simulink model "decentralized_trans"  (R2023b)
settings: Solver=ode45  StartTime=0.0  StopTime=Tf  RelTol=1e-3
undefined symbols (not defined in the file): A_an2, A_an3, Ac_id2, Ac_id3, Ac_mrs2, Ac_mrs3, alpha, b, B_an2, B_an3, Bc_id2, Bc_id3, Bc_mrs2, Bc_mrs3, C2, C3, C_an2, C_an3, C_id2, C_id3, C_opt, Cc_id2, Cc_id3, Cc_mrs2, Cc_mrs3, D_an2, D_an3, Dc_id2, Dc_id3, Dc_mrs2, Dc_mrs3, dx2, dx3, p01, p02, p03, p04, p05, p06, phi02, r_pd1, r_pd2, r_pd3, r_pd4, r_pd5, r_pd6, r_pd_sl1, r_pd_sl2, r_pd_sl3, r_pd_sl4, r_pd_sl5, r_pd_sl6, t1, t2, t3, th, th02, u_max_n1, u_max_n2, u_max_n3 ... (+8)
(part 1 of 2)
settings Model: Creator=lorenzo  LastModifiedBy=lorenzo
settings SolverCC: ZeroCrossControl=DisableAll
settings DebuggingCC: IgnoredZcDiagnostic=none

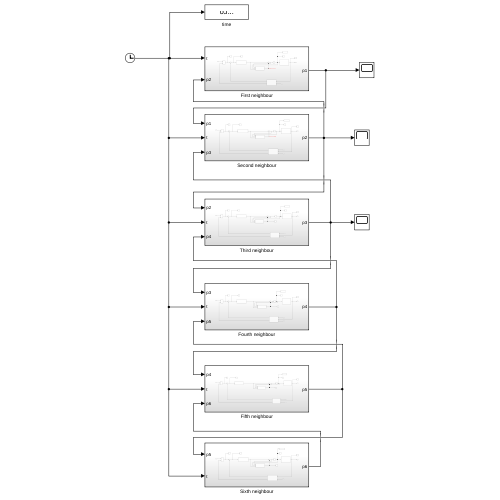
[thumbnail: Simulink's stored preview of the top-level diagram]
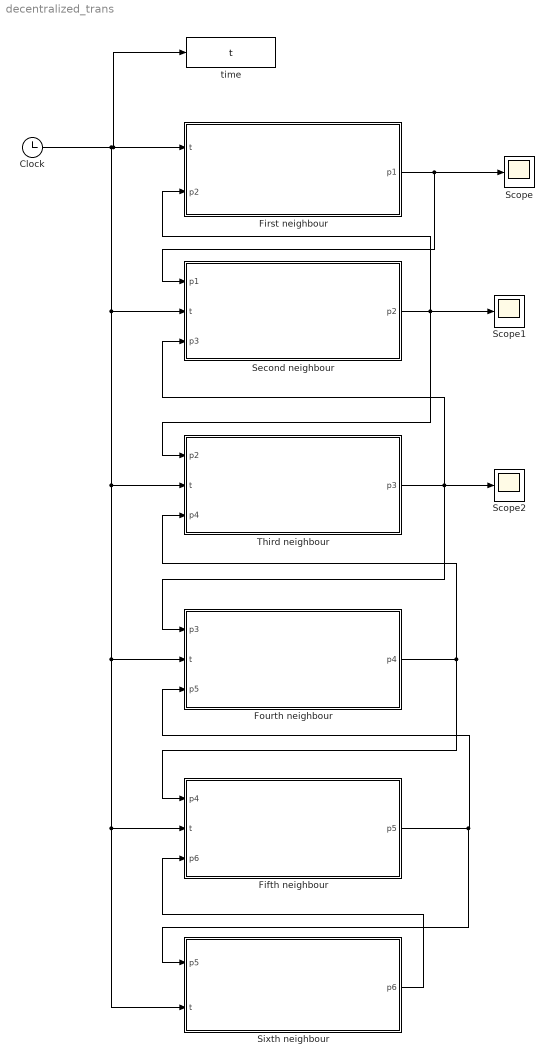
== system decentralized_trans ==
  Clock : Clock
  Fifth neighbour : Subsystem
  First neighbour : Subsystem
  Fourth neighbour : Subsystem
  Scope : Scope
  Scope1 : Scope
  Scope2 : Scope
  Second neighbour : Subsystem
  Sixth neighbour : Subsystem
  Third neighbour : Subsystem
  time : ToWorkspace  VariableName=t  SampleTime=-1
  wires:
  First neighbour/1(p1) -> Second neighbour/1(p1), Scope/1
  Clock/1 -> Sixth neighbour/2(t), Fifth neighbour/2(t), Fourth neighbour/2(t), Third neighbour/2(t), Second neighbour/2(t), First neighbour/1(t), time/1
  Second neighbour/1(p2) -> Scope1/1, First neighbour/2(p2), Third neighbour/1(p2)
  Third neighbour/1(p3) -> Scope2/1, Fourth neighbour/1(p3), Second neighbour/3(p3)
  Fourth neighbour/1(p4) -> Fifth neighbour/1(p4), Third neighbour/3(p4)
  Fifth neighbour/1(p5) -> Sixth neighbour/1(p5), Fourth neighbour/3(p5)
  Sixth neighbour/1(p6) -> Fifth neighbour/3(p6)

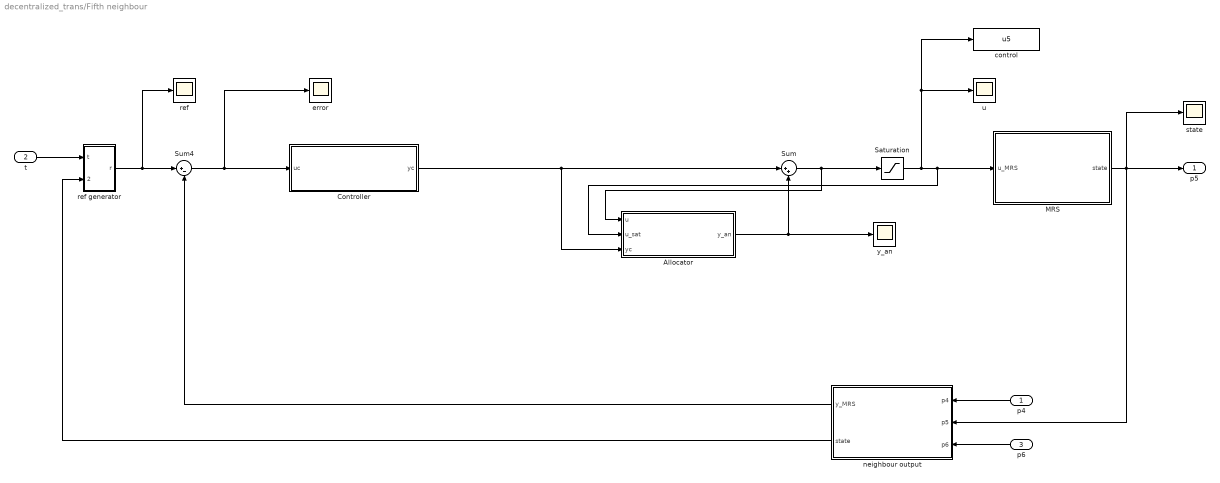
== system decentralized_trans/Fifth neighbour ==
  p4 : Inport
  t : Inport  Port=2
  p6 : Inport  Port=3
  Allocator : Subsystem
  Controller : Subsystem
  MRS : Subsystem
  Saturation : Saturate  UpperLimit=u_max_n5  LowerLimit=-u_max_n5
  Sum : Sum  Inputs=|++
  Sum4 : Sum  Inputs=|+-
  control : ToWorkspace  VariableName=u5  SampleTime=-1
  error : Scope
  neighbour output : Subsystem
  ref : Scope
  ref generator : Subsystem
  state : Scope
  u : Scope
  y_an : Scope
  p5 : Outport
  wires:
  t/1 -> ref generator/1(t)
  Sum4/1 -> error/1, Controller/1(uc)
  MRS/1(state) -> neighbour output/2(p5), state/1, p5/1
  ref generator/1(r) -> ref/1, Sum4/1
  neighbour output/1(y_MRS) -> Sum4/2
  p6/1 -> neighbour output/3(p6)
  neighbour output/2(state) -> ref generator/2(state)
  p4/1 -> neighbour output/1(p4)
  Saturation/1 -> control/1, u/1, Allocator/2(u_sat), MRS/1(u_MRS)
  Sum/1 -> Allocator/1(u), Saturation/1
  Controller/1(yc) -> Allocator/3(yc), Sum/1
  Allocator/1(y_an) -> y_an/1, Sum/2

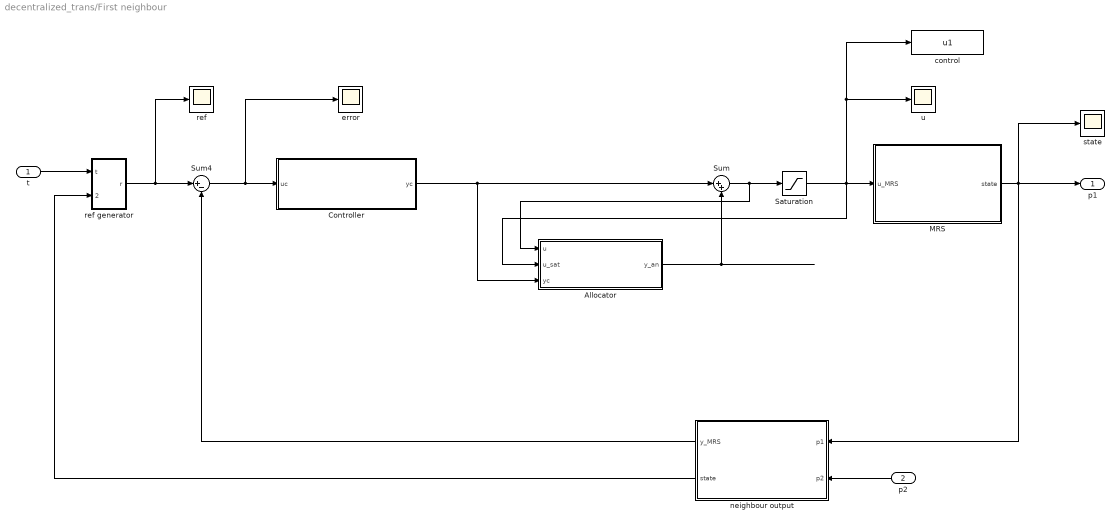
== system decentralized_trans/First neighbour ==
  t : Inport
  p2 : Inport  Port=2
  Allocator : Subsystem
  Controller : Subsystem
  MRS : Subsystem
  Saturation : Saturate  UpperLimit=u_max_n1  LowerLimit=-u_max_n1
  Sum : Sum  Inputs=|++
  Sum4 : Sum  Inputs=|+-
  control : ToWorkspace  VariableName=u1  SampleTime=-1
  error : Scope
  neighbour output : Subsystem
  ref : Scope
  ref generator : Subsystem
  state : Scope
  u : Scope
  p1 : Outport
  wires:
  t/1 -> ref generator/1(t)
  Sum4/1 -> error/1, Controller/1(uc)
  MRS/1(state) -> p1/1, neighbour output/1(p1), state/1
  ref generator/1(r) -> ref/1, Sum4/1
  neighbour output/1(y_MRS) -> Sum4/2
  p2/1 -> neighbour output/2(p2)
  neighbour output/2(state) -> ref generator/2(state)
  Allocator/1(y_an) -> Sum/2
  Sum/1 -> Allocator/1(u), Saturation/1
  Controller/1(yc) -> Allocator/3(yc), Sum/1
  Saturation/1 -> MRS/1(u_MRS), control/1, u/1, Allocator/2(u_sat)

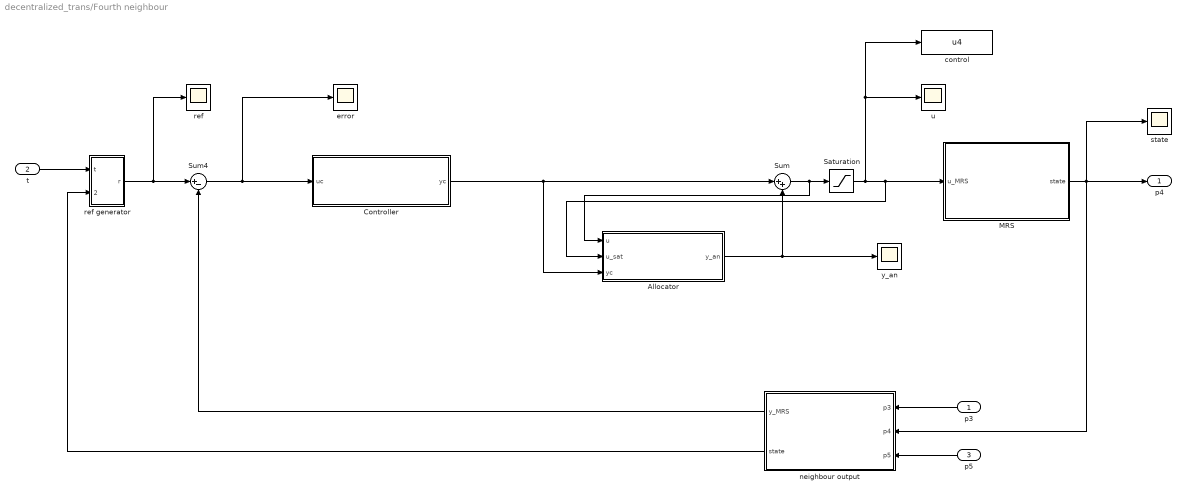
== system decentralized_trans/Fourth neighbour ==
  p3 : Inport
  t : Inport  Port=2
  p5 : Inport  Port=3
  Allocator : Subsystem
  Controller : Subsystem
  MRS : Subsystem
  Saturation : Saturate  UpperLimit=u_max_n4  LowerLimit=-u_max_n4
  Sum : Sum  Inputs=|++
  Sum4 : Sum  Inputs=|+-
  control : ToWorkspace  VariableName=u4  SampleTime=-1
  error : Scope
  neighbour output : Subsystem
  ref : Scope
  ref generator : Subsystem
  state : Scope
  u : Scope
  y_an : Scope
  p4 : Outport
  wires:
  t/1 -> ref generator/1(t)
  Sum4/1 -> error/1, Controller/1(uc)
  MRS/1(state) -> neighbour output/2(p4), state/1, p4/1
  ref generator/1(r) -> ref/1, Sum4/1
  neighbour output/1(y_MRS) -> Sum4/2
  p5/1 -> neighbour output/3(p5)
  neighbour output/2(state) -> ref generator/2(state)
  p3/1 -> neighbour output/1(p3)
  Saturation/1 -> control/1, u/1, Allocator/2(u_sat), MRS/1(u_MRS)
  Sum/1 -> Allocator/1(u), Saturation/1
  Controller/1(yc) -> Allocator/3(yc), Sum/1
  Allocator/1(y_an) -> y_an/1, Sum/2

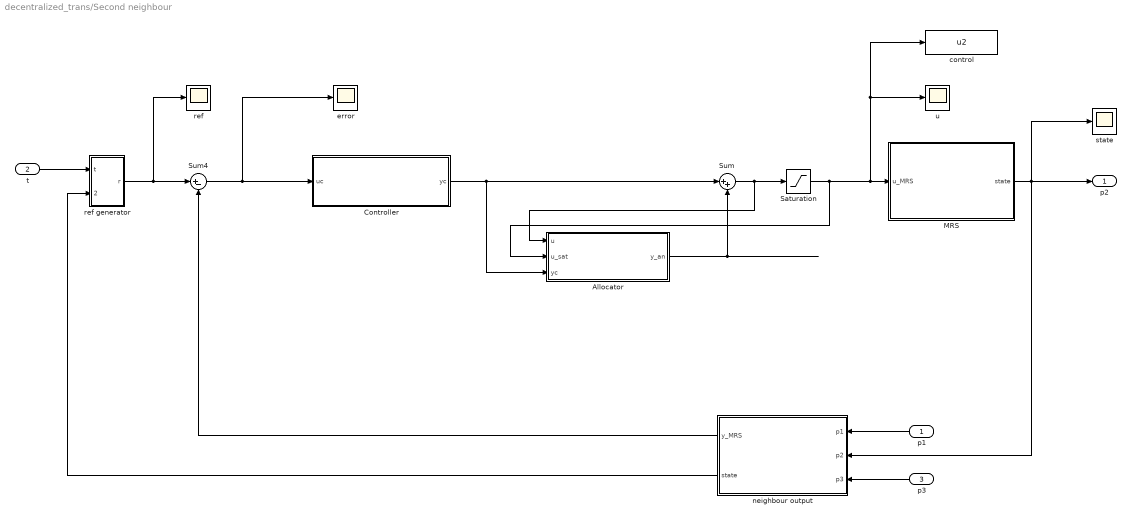
== system decentralized_trans/Second neighbour ==
  p1 : Inport
  t : Inport  Port=2
  p3 : Inport  Port=3
  Allocator : Subsystem
  Controller : Subsystem
  MRS : Subsystem
  Saturation : Saturate  UpperLimit=u_max_n2  LowerLimit=-u_max_n2
  Sum : Sum  Inputs=|++
  Sum4 : Sum  Inputs=|+-
  control : ToWorkspace  VariableName=u2  SampleTime=-1
  error : Scope
  neighbour output : Subsystem
  ref : Scope
  ref generator : Subsystem
  state : Scope
  u : Scope
  p2 : Outport
  wires:
  t/1 -> ref generator/1(t)
  Sum4/1 -> error/1, Controller/1(uc)
  MRS/1(state) -> neighbour output/2(p2), state/1, p2/1
  ref generator/1(r) -> ref/1, Sum4/1
  neighbour output/1(y_MRS) -> Sum4/2
  p3/1 -> neighbour output/3(p3)
  neighbour output/2(state) -> ref generator/2(state)
  p1/1 -> neighbour output/1(p1)
  Allocator/1(y_an) -> Sum/2
  Controller/1(yc) -> Allocator/3(yc), Sum/1
  Sum/1 -> Allocator/1(u), Saturation/1
  Saturation/1 -> MRS/1(u_MRS), control/1, u/1, Allocator/2(u_sat)

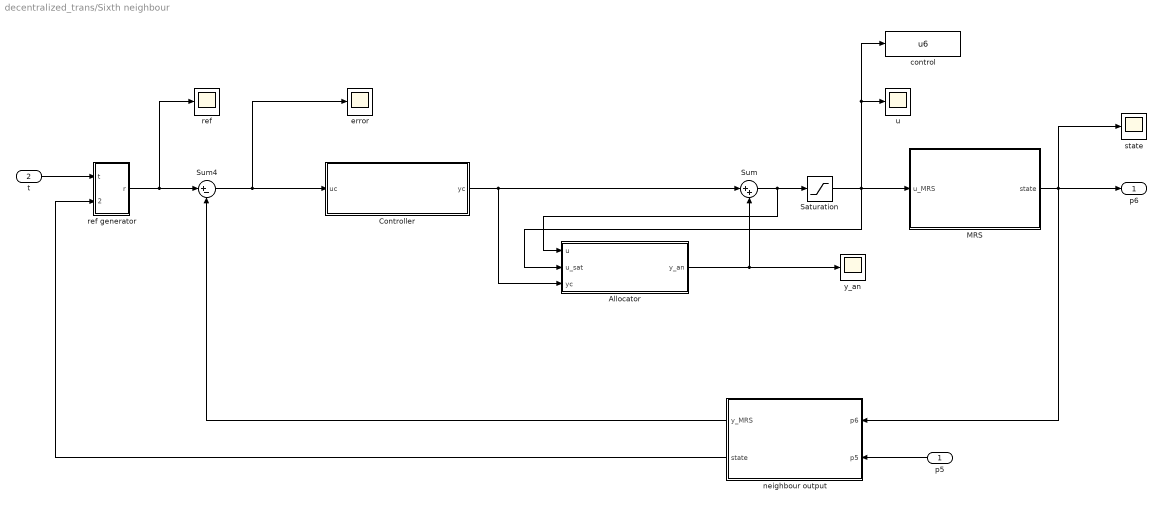
== system decentralized_trans/Sixth neighbour ==
  p5 : Inport
  t : Inport  Port=2
  Allocator : Subsystem
  Controller : Subsystem
  MRS : Subsystem
  Saturation : Saturate  UpperLimit=u_max_n6  LowerLimit=-u_max_n6
  Sum : Sum  Inputs=|++
  Sum4 : Sum  Inputs=|+-
  control : ToWorkspace  VariableName=u6  SampleTime=-1
  error : Scope
  neighbour output : Subsystem
  ref : Scope
  ref generator : Subsystem
  state : Scope
  u : Scope
  y_an : Scope
  p6 : Outport
  wires:
  t/1 -> ref generator/1(t)
  Sum4/1 -> error/1, Controller/1(uc)
  MRS/1(state) -> neighbour output/1(p6), state/1, p6/1
  ref generator/1(r) -> ref/1, Sum4/1
  neighbour output/1(y_MRS) -> Sum4/2
  p5/1 -> neighbour output/2(p5)
  neighbour output/2(state) -> ref generator/2(state)
  Allocator/1(y_an) -> y_an/1, Sum/2
  Controller/1(yc) -> Allocator/3(yc), Sum/1
  Sum/1 -> Allocator/1(u), Saturation/1
  Saturation/1 -> control/1, u/1, Allocator/2(u_sat), MRS/1(u_MRS)

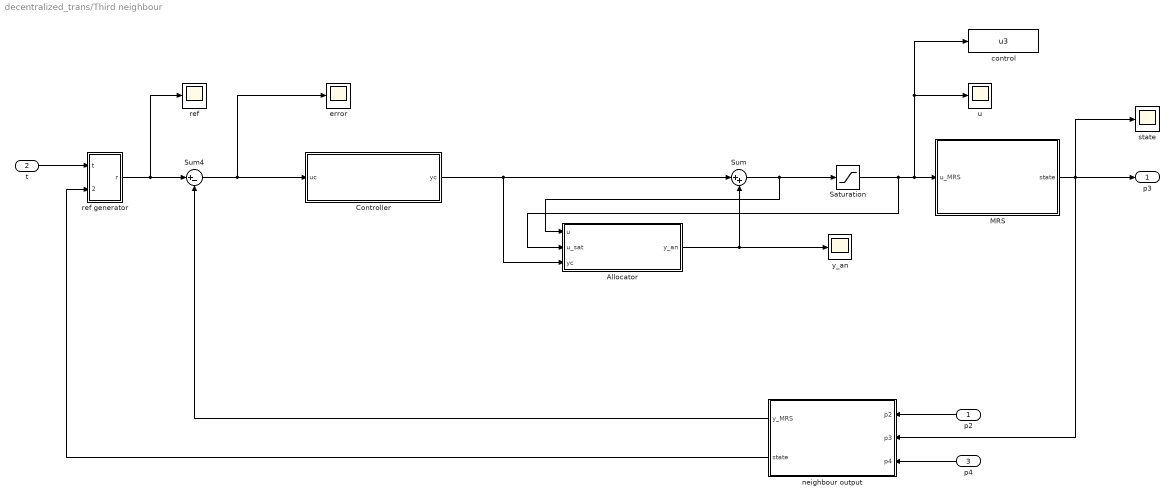
== system decentralized_trans/Third neighbour ==
  p2 : Inport
  t : Inport  Port=2
  p4 : Inport  Port=3
  Allocator : Subsystem
  Controller : Subsystem
  MRS : Subsystem
  Saturation : Saturate  UpperLimit=u_max_n3  LowerLimit=-u_max_n3
  Sum : Sum  Inputs=|++
  Sum4 : Sum  Inputs=|+-
  control : ToWorkspace  VariableName=u3  SampleTime=-1
  error : Scope
  neighbour output : Subsystem
  ref : Scope
  ref generator : Subsystem
  state : Scope
  u : Scope
  y_an : Scope
  p3 : Outport
  wires:
  t/1 -> ref generator/1(t)
  Sum4/1 -> error/1, Controller/1(uc)
  MRS/1(state) -> neighbour output/2(p3), state/1, p3/1
  ref generator/1(r) -> ref/1, Sum4/1
  neighbour output/1(y_MRS) -> Sum4/2
  p4/1 -> neighbour output/3(p4)
  neighbour output/2(state) -> ref generator/2(state)
  p2/1 -> neighbour output/1(p2)
  Saturation/1 -> MRS/1(u_MRS), control/1, u/1, Allocator/2(u_sat)
  Sum/1 -> Allocator/1(u), Saturation/1
  Controller/1(yc) -> Allocator/3(yc), Sum/1
  Allocator/1(y_an) -> y_an/1, Sum/2

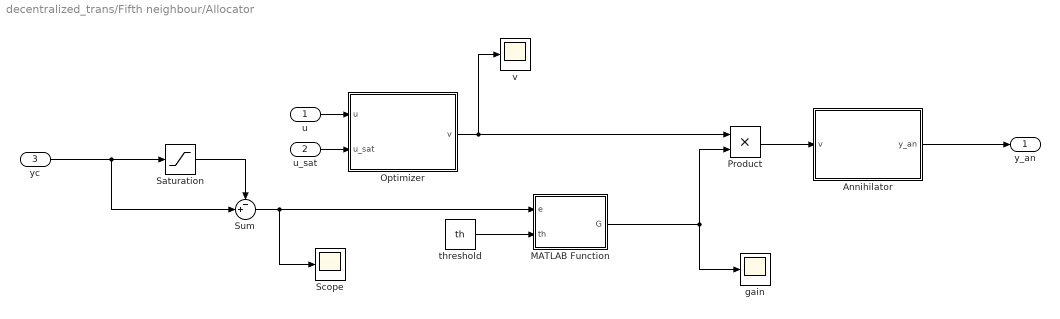
== system decentralized_trans/Fifth neighbour/Allocator ==
  u : Inport
  u_sat : Inport  Port=2
  yc : Inport  Port=3
  Annihilator : Subsystem
  MATLAB Function : MATLAB Function  TreatAsAtomicUnit=on
  Optimizer : Subsystem
  Product : Product
  Saturation : Saturate  UpperLimit=u_max_n5  LowerLimit=-u_max_n5
  Scope : Scope
  Sum : Sum  Inputs=-+|
  gain : Scope
  threshold : Constant  Value=th
  v : Scope
  y_an : Outport
  wires:
  threshold/1 -> MATLAB Function/2(th)
  Optimizer/1(v) -> Product/1, v/1
  u_sat/1 -> Optimizer/2(u_sat)
  MATLAB Function/1(G) -> gain/1, Product/2
  u/1 -> Optimizer/1(u)
  Annihilator/1(y_an) -> y_an/1
  Product/1 -> Annihilator/1(v)
  Saturation/1 -> Sum/1
  Sum/1 -> Scope/1, MATLAB Function/1(e)
  yc/1 -> Sum/2, Saturation/1

== system decentralized_trans/Fifth neighbour/Controller ==
  uc : Inport
  Clock1 : Clock
  Controller formation : Subsystem
  Controller line follow : Subsystem
  MATLAB Function : MATLAB Function  TreatAsAtomicUnit=on
  MATLAB Function1 : MATLAB Function  TreatAsAtomicUnit=on
  Scope : Scope
  t1 : Constant  Value=t1  VectorParams1D=off
  t2 : Constant  Value=t2  VectorParams1D=off
  t3 : Constant  Value=t3  VectorParams1D=off
  yc : Outport
  wires:
  uc/1 -> Controller formation/1(uc), Controller line follow/1(uc)
  Clock1/1 -> MATLAB Function1/1(t), MATLAB Function/2(t)
  Controller line follow/1(u) -> MATLAB Function/1(u_lf)
  Controller formation/1(u) -> MATLAB Function/3(u_f)
  t1/1 -> MATLAB Function1/2(t1), MATLAB Function/4(t1)
  t3/1 -> MATLAB Function1/4(t3), MATLAB Function/6(t3)
  MATLAB Function/1(yc) -> yc/1
  t2/1 -> MATLAB Function1/3(t2), MATLAB Function/5(t2)
  MATLAB Function1/1(y) -> Scope/1, Controller line follow/2(y), Controller formation/2(y)

== system decentralized_trans/Fifth neighbour/MRS ==
  u_MRS : Inport
  Constant : Constant  Value=b
  Integrator : Integrator  InitialCondition=p05
  Integrator1 : Integrator  InitialCondition=th02
  Integrator2 : Integrator  InitialCondition=phi02
  MATLAB Function : MATLAB Function  TreatAsAtomicUnit=on
  Scope : Scope
  Scope1 : Scope
  theta : ToWorkspace  VariableName=theta5  SampleTime=-1
  y : ToWorkspace  VariableName=y5  SampleTime=-1
  state : Outport
  wires:
  u_MRS/1 -> MATLAB Function/1(u)
  Constant/1 -> MATLAB Function/2(b)
  MATLAB Function/2(dth) -> Integrator1/1
  MATLAB Function/1(dp) -> Integrator/1
  Integrator1/1 -> MATLAB Function/3(th), Scope/1, theta/1
  MATLAB Function/3(dphi) -> Integrator2/1
  Integrator2/1 -> Scope1/1, MATLAB Function/4(phi)
  Integrator/1 -> y/1, state/1

== system decentralized_trans/Fifth neighbour/neighbour output ==
  p4 : Inport
  p5 : Inport  Port=2
  p6 : Inport  Port=3
  C : Gain  Gain=C3  Multiplication=Matrix(K*u) (u vector)
  C_id : Gain  Gain=C_id3  Multiplication=Matrix(K*u) (u vector)
  Clock : Clock
  MATLAB Function : MATLAB Function  TreatAsAtomicUnit=on
  MATLAB Function1 : MATLAB Function  TreatAsAtomicUnit=on
  t1 : Constant  Value=t1  VectorParams1D=off
  t2 : Constant  Value=t2  VectorParams1D=off
  t3 : Constant  Value=t3  VectorParams1D=off
  y_MRS : Outport
  state : Outport  Port=2
  wires:
  t2/1 -> MATLAB Function1/5(t2)
  C/1 -> MATLAB Function1/3(y_f)
  Clock/1 -> MATLAB Function1/2(t)
  t3/1 -> MATLAB Function1/6(t3)
  C_id/1 -> MATLAB Function1/1(y_lf)
  MATLAB Function1/1(y_MRS) -> y_MRS/1
  t1/1 -> MATLAB Function1/4(t1)
  MATLAB Function/1(yn) -> state/1, C/1, C_id/1
  p6/1 -> MATLAB Function/3(y3)
  p5/1 -> MATLAB Function/2(y2)
  p4/1 -> MATLAB Function/1(y1)

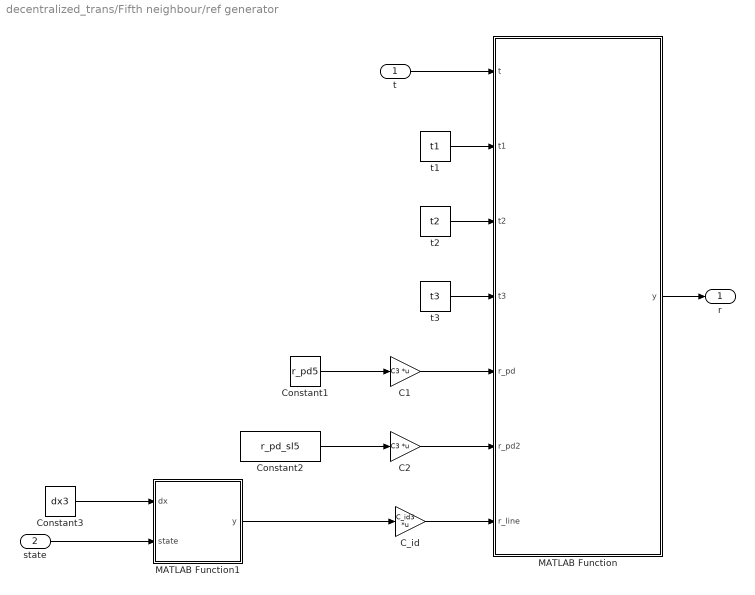
== system decentralized_trans/Fifth neighbour/ref generator ==
  t : Inport
  state : Inport  Port=2
  C1 : Gain  Gain=C3  Multiplication=Matrix(K*u) (u vector)
  C2 : Gain  Gain=C3  Multiplication=Matrix(K*u) (u vector)
  C_id : Gain  Gain=C_id3  Multiplication=Matrix(K*u) (u vector)
  Constant1 : Constant  Value=r_pd5  VectorParams1D=off
  Constant2 : Constant  Value=r_pd_sl5  VectorParams1D=off
  Constant3 : Constant  Value=dx3
  MATLAB Function : MATLAB Function  TreatAsAtomicUnit=on
  MATLAB Function1 : MATLAB Function  TreatAsAtomicUnit=on
  t1 : Constant  Value=t1  VectorParams1D=off
  t2 : Constant  Value=t2  VectorParams1D=off
  t3 : Constant  Value=t3  VectorParams1D=off
  r : Outport
  wires:
  t/1 -> MATLAB Function/1(t)
  t1/1 -> MATLAB Function/2(t1)
  t2/1 -> MATLAB Function/3(t2)
  t3/1 -> MATLAB Function/4(t3)
  Constant2/1 -> C2/1
  C2/1 -> MATLAB Function/6(r_pd2)
  Constant1/1 -> C1/1
  C1/1 -> MATLAB Function/5(r_pd)
  C_id/1 -> MATLAB Function/7(r_line)
  MATLAB Function/1(y) -> r/1
  Constant3/1 -> MATLAB Function1/1(dx)
  state/1 -> MATLAB Function1/2(state)
  MATLAB Function1/1(y) -> C_id/1

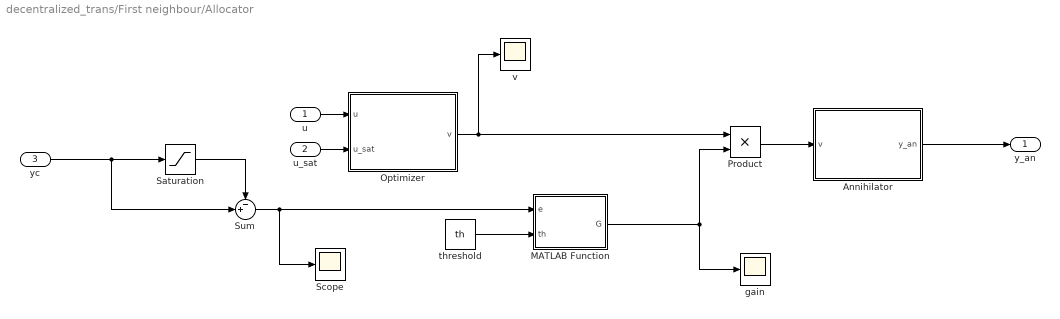
== system decentralized_trans/First neighbour/Allocator ==
  u : Inport
  u_sat : Inport  Port=2
  yc : Inport  Port=3
  Annihilator : Subsystem
  MATLAB Function : MATLAB Function  TreatAsAtomicUnit=on
  Optimizer : Subsystem
  Product : Product
  Saturation : Saturate  UpperLimit=u_max_n1  LowerLimit=-u_max_n1
  Scope : Scope
  Sum : Sum  Inputs=-+|
  gain : Scope
  threshold : Constant  Value=th
  v : Scope
  y_an : Outport
  wires:
  threshold/1 -> MATLAB Function/2(th)
  Optimizer/1(v) -> Product/1, v/1
  u_sat/1 -> Optimizer/2(u_sat)
  MATLAB Function/1(G) -> gain/1, Product/2
  u/1 -> Optimizer/1(u)
  Annihilator/1(y_an) -> y_an/1
  Product/1 -> Annihilator/1(v)
  Saturation/1 -> Sum/1
  Sum/1 -> Scope/1, MATLAB Function/1(e)
  yc/1 -> Sum/2, Saturation/1

== system decentralized_trans/First neighbour/Controller ==
  uc : Inport
  Clock1 : Clock
  Controller formation : Subsystem
  Controller line follow : Subsystem
  MATLAB Function : MATLAB Function  TreatAsAtomicUnit=on
  MATLAB Function1 : MATLAB Function  TreatAsAtomicUnit=on
  Scope : Scope
  t1 : Constant  Value=t1  VectorParams1D=off
  t2 : Constant  Value=t2  VectorParams1D=off
  t3 : Constant  Value=t3  VectorParams1D=off
  yc : Outport
  wires:
  uc/1 -> Controller formation/1(uc), Controller line follow/1(uc)
  Clock1/1 -> MATLAB Function1/1(t), MATLAB Function/2(t)
  Controller line follow/1(u) -> MATLAB Function/1(u_lf)
  Controller formation/1(u) -> MATLAB Function/3(u_f)
  t1/1 -> MATLAB Function1/2(t1), MATLAB Function/4(t1)
  t3/1 -> MATLAB Function1/4(t3), MATLAB Function/6(t3)
  MATLAB Function/1(yc) -> yc/1
  t2/1 -> MATLAB Function1/3(t2), MATLAB Function/5(t2)
  MATLAB Function1/1(y) -> Scope/1, Controller line follow/2(y), Controller formation/2(y)

== system decentralized_trans/First neighbour/MRS ==
  u_MRS : Inport
  Constant : Constant  Value=b
  Integrator : Integrator  InitialCondition=p01
  Integrator1 : Integrator  InitialCondition=th02
  Integrator2 : Integrator  InitialCondition=phi02
  MATLAB Function : MATLAB Function  TreatAsAtomicUnit=on
  Scope : Scope
  Scope1 : Scope
  theta : ToWorkspace  VariableName=theta1  SampleTime=-1
  y : ToWorkspace  VariableName=y1  SampleTime=-1
  state : Outport
  wires:
  u_MRS/1 -> MATLAB Function/1(u)
  Constant/1 -> MATLAB Function/2(b)
  MATLAB Function/2(dth) -> Integrator1/1
  MATLAB Function/1(dp) -> Integrator/1
  Integrator1/1 -> MATLAB Function/3(th), Scope/1, theta/1
  MATLAB Function/3(dphi) -> Integrator2/1
  Integrator2/1 -> Scope1/1, MATLAB Function/4(phi)
  Integrator/1 -> y/1, state/1

== system decentralized_trans/First neighbour/neighbour output ==
  p1 : Inport
  p2 : Inport  Port=2
  C : Gain  Gain=C2  Multiplication=Matrix(K*u) (u vector)
  C_id : Gain  Gain=C_id2  Multiplication=Matrix(K*u) (u vector)
  Clock : Clock
  MATLAB Function : MATLAB Function  TreatAsAtomicUnit=on
  MATLAB Function1 : MATLAB Function  TreatAsAtomicUnit=on
  t1 : Constant  Value=t1  VectorParams1D=off
  t2 : Constant  Value=t2  VectorParams1D=off
  t3 : Constant  Value=t3  VectorParams1D=off
  y_MRS : Outport
  state : Outport  Port=2
  wires:
  t2/1 -> MATLAB Function1/5(t2)
  C/1 -> MATLAB Function1/3(y_f)
  Clock/1 -> MATLAB Function1/2(t)
  t3/1 -> MATLAB Function1/6(t3)
  C_id/1 -> MATLAB Function1/1(y_lf)
  MATLAB Function1/1(y_MRS) -> y_MRS/1
  t1/1 -> MATLAB Function1/4(t1)
  p1/1 -> MATLAB Function/1(y1)
  p2/1 -> MATLAB Function/2(y2)
  MATLAB Function/1(yn) -> state/1, C/1, C_id/1

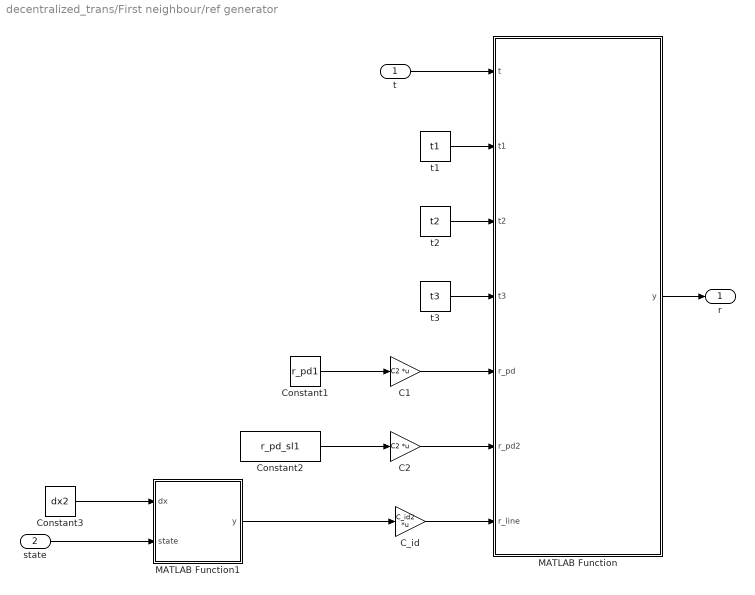
== system decentralized_trans/First neighbour/ref generator ==
  t : Inport
  state : Inport  Port=2
  C1 : Gain  Gain=C2  Multiplication=Matrix(K*u) (u vector)
  C2 : Gain  Gain=C2  Multiplication=Matrix(K*u) (u vector)
  C_id : Gain  Gain=C_id2  Multiplication=Matrix(K*u) (u vector)
  Constant1 : Constant  Value=r_pd1  VectorParams1D=off
  Constant2 : Constant  Value=r_pd_sl1  VectorParams1D=off
  Constant3 : Constant  Value=dx2
  MATLAB Function : MATLAB Function  TreatAsAtomicUnit=on
  MATLAB Function1 : MATLAB Function  TreatAsAtomicUnit=on
  t1 : Constant  Value=t1  VectorParams1D=off
  t2 : Constant  Value=t2  VectorParams1D=off
  t3 : Constant  Value=t3  VectorParams1D=off
  r : Outport
  wires:
  t/1 -> MATLAB Function/1(t)
  t1/1 -> MATLAB Function/2(t1)
  t2/1 -> MATLAB Function/3(t2)
  t3/1 -> MATLAB Function/4(t3)
  Constant2/1 -> C2/1
  C2/1 -> MATLAB Function/6(r_pd2)
  Constant1/1 -> C1/1
  C1/1 -> MATLAB Function/5(r_pd)
  C_id/1 -> MATLAB Function/7(r_line)
  MATLAB Function/1(y) -> r/1
  Constant3/1 -> MATLAB Function1/1(dx)
  state/1 -> MATLAB Function1/2(state)
  MATLAB Function1/1(y) -> C_id/1

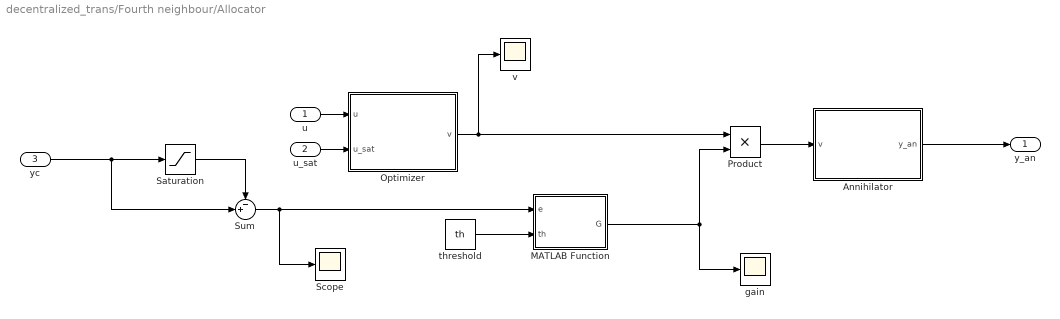
== system decentralized_trans/Fourth neighbour/Allocator ==
  u : Inport
  u_sat : Inport  Port=2
  yc : Inport  Port=3
  Annihilator : Subsystem
  MATLAB Function : MATLAB Function  TreatAsAtomicUnit=on
  Optimizer : Subsystem
  Product : Product
  Saturation : Saturate  UpperLimit=u_max_n4  LowerLimit=-u_max_n4
  Scope : Scope
  Sum : Sum  Inputs=-+|
  gain : Scope
  threshold : Constant  Value=th
  v : Scope
  y_an : Outport
  wires:
  threshold/1 -> MATLAB Function/2(th)
  Optimizer/1(v) -> Product/1, v/1
  u_sat/1 -> Optimizer/2(u_sat)
  MATLAB Function/1(G) -> gain/1, Product/2
  u/1 -> Optimizer/1(u)
  Annihilator/1(y_an) -> y_an/1
  Product/1 -> Annihilator/1(v)
  Saturation/1 -> Sum/1
  Sum/1 -> Scope/1, MATLAB Function/1(e)
  yc/1 -> Sum/2, Saturation/1

== system decentralized_trans/Fourth neighbour/Controller ==
  uc : Inport
  Clock1 : Clock
  Controller formation : Subsystem
  Controller line follow : Subsystem
  MATLAB Function : MATLAB Function  TreatAsAtomicUnit=on
  MATLAB Function1 : MATLAB Function  TreatAsAtomicUnit=on
  Scope : Scope
  t1 : Constant  Value=t1  VectorParams1D=off
  t2 : Constant  Value=t2  VectorParams1D=off
  t3 : Constant  Value=t3  VectorParams1D=off
  yc : Outport
  wires:
  uc/1 -> Controller formation/1(uc), Controller line follow/1(uc)
  Clock1/1 -> MATLAB Function1/1(t), MATLAB Function/2(t)
  Controller line follow/1(u) -> MATLAB Function/1(u_lf)
  Controller formation/1(u) -> MATLAB Function/3(u_f)
  t1/1 -> MATLAB Function1/2(t1), MATLAB Function/4(t1)
  t3/1 -> MATLAB Function1/4(t3), MATLAB Function/6(t3)
  MATLAB Function/1(yc) -> yc/1
  t2/1 -> MATLAB Function1/3(t2), MATLAB Function/5(t2)
  MATLAB Function1/1(y) -> Scope/1, Controller line follow/2(y), Controller formation/2(y)

== system decentralized_trans/Fourth neighbour/MRS ==
  u_MRS : Inport
  Constant : Constant  Value=b
  Integrator : Integrator  InitialCondition=p04
  Integrator1 : Integrator  InitialCondition=th02
  Integrator2 : Integrator  InitialCondition=phi02
  MATLAB Function : MATLAB Function  TreatAsAtomicUnit=on
  Scope : Scope
  Scope1 : Scope
  theta : ToWorkspace  VariableName=theta4  SampleTime=-1
  y : ToWorkspace  VariableName=y4  SampleTime=-1
  state : Outport
  wires:
  u_MRS/1 -> MATLAB Function/1(u)
  Constant/1 -> MATLAB Function/2(b)
  MATLAB Function/2(dth) -> Integrator1/1
  MATLAB Function/1(dp) -> Integrator/1
  Integrator1/1 -> MATLAB Function/3(th), Scope/1, theta/1
  MATLAB Function/3(dphi) -> Integrator2/1
  Integrator2/1 -> Scope1/1, MATLAB Function/4(phi)
  Integrator/1 -> y/1, state/1

== system decentralized_trans/Fourth neighbour/neighbour output ==
  p3 : Inport
  p4 : Inport  Port=2
  p5 : Inport  Port=3
  C : Gain  Gain=C3  Multiplication=Matrix(K*u) (u vector)
  C_id : Gain  Gain=C_id3  Multiplication=Matrix(K*u) (u vector)
  Clock : Clock
  MATLAB Function : MATLAB Function  TreatAsAtomicUnit=on
  MATLAB Function1 : MATLAB Function  TreatAsAtomicUnit=on
  t1 : Constant  Value=t1  VectorParams1D=off
  t2 : Constant  Value=t2  VectorParams1D=off
  t3 : Constant  Value=t3  VectorParams1D=off
  y_MRS : Outport
  state : Outport  Port=2
  wires:
  t2/1 -> MATLAB Function1/5(t2)
  C/1 -> MATLAB Function1/3(y_f)
  Clock/1 -> MATLAB Function1/2(t)
  t3/1 -> MATLAB Function1/6(t3)
  C_id/1 -> MATLAB Function1/1(y_lf)
  MATLAB Function1/1(y_MRS) -> y_MRS/1
  t1/1 -> MATLAB Function1/4(t1)
  MATLAB Function/1(yn) -> state/1, C/1, C_id/1
  p5/1 -> MATLAB Function/3(y3)
  p4/1 -> MATLAB Function/2(y2)
  p3/1 -> MATLAB Function/1(y1)

== system decentralized_trans/Fourth neighbour/ref generator ==
  t : Inport
  state : Inport  Port=2
  C1 : Gain  Gain=C3  Multiplication=Matrix(K*u) (u vector)
  C2 : Gain  Gain=C3  Multiplication=Matrix(K*u) (u vector)
  C_id : Gain  Gain=C_id3  Multiplication=Matrix(K*u) (u vector)
  Constant1 : Constant  Value=r_pd4  VectorParams1D=off
  Constant2 : Constant  Value=r_pd_sl4  VectorParams1D=off
  Constant3 : Constant  Value=dx3
  MATLAB Function : MATLAB Function  TreatAsAtomicUnit=on
  MATLAB Function1 : MATLAB Function  TreatAsAtomicUnit=on
  t1 : Constant  Value=t1  VectorParams1D=off
  t2 : Constant  Value=t2  VectorParams1D=off
  t3 : Constant  Value=t3  VectorParams1D=off
  r : Outport
  wires:
  t/1 -> MATLAB Function/1(t)
  t1/1 -> MATLAB Function/2(t1)
  t2/1 -> MATLAB Function/3(t2)
  t3/1 -> MATLAB Function/4(t3)
  Constant2/1 -> C2/1
  C2/1 -> MATLAB Function/6(r_pd2)
  Constant1/1 -> C1/1
  C1/1 -> MATLAB Function/5(r_pd)
  C_id/1 -> MATLAB Function/7(r_line)
  MATLAB Function/1(y) -> r/1
  Constant3/1 -> MATLAB Function1/1(dx)
  state/1 -> MATLAB Function1/2(state)
  MATLAB Function1/1(y) -> C_id/1

== system decentralized_trans/Second neighbour/Allocator ==
  u : Inport
  u_sat : Inport  Port=2
  yc : Inport  Port=3
  Annihilator : Subsystem
  MATLAB Function : MATLAB Function  TreatAsAtomicUnit=on
  Optimizer : Subsystem
  Product : Product
  Saturation : Saturate  UpperLimit=u_max_n2  LowerLimit=-u_max_n2
  Scope : Scope
  Sum : Sum  Inputs=-+|
  gain : Scope
  threshold : Constant  Value=th
  v : Scope
  y_an : Outport
  wires:
  threshold/1 -> MATLAB Function/2(th)
  Optimizer/1(v) -> Product/1, v/1
  u_sat/1 -> Optimizer/2(u_sat)
  MATLAB Function/1(G) -> gain/1, Product/2
  u/1 -> Optimizer/1(u)
  Annihilator/1(y_an) -> y_an/1
  Product/1 -> Annihilator/1(v)
  Saturation/1 -> Sum/1
  Sum/1 -> Scope/1, MATLAB Function/1(e)
  yc/1 -> Sum/2, Saturation/1

== system decentralized_trans/Second neighbour/Controller ==
  uc : Inport
  Clock1 : Clock
  Controller formation : Subsystem
  Controller line follow : Subsystem
  MATLAB Function : MATLAB Function  TreatAsAtomicUnit=on
  MATLAB Function1 : MATLAB Function  TreatAsAtomicUnit=on
  Scope : Scope
  t1 : Constant  Value=t1  VectorParams1D=off
  t2 : Constant  Value=t2  VectorParams1D=off
  t3 : Constant  Value=t3  VectorParams1D=off
  yc : Outport
  wires:
  uc/1 -> Controller formation/1(uc), Controller line follow/1(uc)
  Clock1/1 -> MATLAB Function1/1(t), MATLAB Function/2(t)
  Controller line follow/1(u) -> MATLAB Function/1(u_lf)
  Controller formation/1(u) -> MATLAB Function/3(u_f)
  t1/1 -> MATLAB Function1/2(t1), MATLAB Function/4(t1)
  t3/1 -> MATLAB Function1/4(t3), MATLAB Function/6(t3)
  MATLAB Function/1(yc) -> yc/1
  t2/1 -> MATLAB Function1/3(t2), MATLAB Function/5(t2)
  MATLAB Function1/1(y) -> Scope/1, Controller line follow/2(y), Controller formation/2(y)

== system decentralized_trans/Second neighbour/MRS ==
  u_MRS : Inport
  Constant : Constant  Value=b
  Integrator : Integrator  InitialCondition=p02
  Integrator1 : Integrator  InitialCondition=th02
  Integrator2 : Integrator  InitialCondition=phi02
  MATLAB Function : MATLAB Function  TreatAsAtomicUnit=on
  Scope : Scope
  Scope1 : Scope
  theta : ToWorkspace  VariableName=theta2  SampleTime=-1
  y : ToWorkspace  VariableName=y2  SampleTime=-1
  state : Outport
  wires:
  u_MRS/1 -> MATLAB Function/1(u)
  Constant/1 -> MATLAB Function/2(b)
  MATLAB Function/2(dth) -> Integrator1/1
  MATLAB Function/1(dp) -> Integrator/1
  Integrator1/1 -> MATLAB Function/3(th), Scope/1, theta/1
  MATLAB Function/3(dphi) -> Integrator2/1
  Integrator2/1 -> Scope1/1, MATLAB Function/4(phi)
  Integrator/1 -> y/1, state/1

== system decentralized_trans/Second neighbour/neighbour output ==
  p1 : Inport
  p2 : Inport  Port=2
  p3 : Inport  Port=3
  C : Gain  Gain=C3  Multiplication=Matrix(K*u) (u vector)
  C_id : Gain  Gain=C_id3  Multiplication=Matrix(K*u) (u vector)
  Clock : Clock
  MATLAB Function : MATLAB Function  TreatAsAtomicUnit=on
  MATLAB Function1 : MATLAB Function  TreatAsAtomicUnit=on
  t1 : Constant  Value=t1  VectorParams1D=off
  t2 : Constant  Value=t2  VectorParams1D=off
  t3 : Constant  Value=t3  VectorParams1D=off
  y_MRS : Outport
  state : Outport  Port=2
  wires:
  t2/1 -> MATLAB Function1/5(t2)
  C/1 -> MATLAB Function1/3(y_f)
  Clock/1 -> MATLAB Function1/2(t)
  t3/1 -> MATLAB Function1/6(t3)
  C_id/1 -> MATLAB Function1/1(y_lf)
  MATLAB Function1/1(y_MRS) -> y_MRS/1
  t1/1 -> MATLAB Function1/4(t1)
  MATLAB Function/1(yn) -> state/1, C/1, C_id/1
  p3/1 -> MATLAB Function/3(y3)
  p2/1 -> MATLAB Function/2(y2)
  p1/1 -> MATLAB Function/1(y1)

== system decentralized_trans/Second neighbour/ref generator ==
  t : Inport
  state : Inport  Port=2
  C1 : Gain  Gain=C3  Multiplication=Matrix(K*u) (u vector)
  C2 : Gain  Gain=C3  Multiplication=Matrix(K*u) (u vector)
  C_id : Gain  Gain=C_id3  Multiplication=Matrix(K*u) (u vector)
  Constant1 : Constant  Value=r_pd2  VectorParams1D=off
  Constant2 : Constant  Value=r_pd_sl2  VectorParams1D=off
  Constant3 : Constant  Value=dx3
  MATLAB Function : MATLAB Function  TreatAsAtomicUnit=on
  MATLAB Function1 : MATLAB Function  TreatAsAtomicUnit=on
  t1 : Constant  Value=t1  VectorParams1D=off
  t2 : Constant  Value=t2  VectorParams1D=off
  t3 : Constant  Value=t3  VectorParams1D=off
  r : Outport
  wires:
  t/1 -> MATLAB Function/1(t)
  t1/1 -> MATLAB Function/2(t1)
  t2/1 -> MATLAB Function/3(t2)
  t3/1 -> MATLAB Function/4(t3)
  Constant2/1 -> C2/1
  C2/1 -> MATLAB Function/6(r_pd2)
  Constant1/1 -> C1/1
  C1/1 -> MATLAB Function/5(r_pd)
  C_id/1 -> MATLAB Function/7(r_line)
  MATLAB Function/1(y) -> r/1
  Constant3/1 -> MATLAB Function1/1(dx)
  state/1 -> MATLAB Function1/2(state)
  MATLAB Function1/1(y) -> C_id/1

== system decentralized_trans/Sixth neighbour/Allocator ==
  u : Inport
  u_sat : Inport  Port=2
  yc : Inport  Port=3
  Annihilator : Subsystem
  MATLAB Function : MATLAB Function  TreatAsAtomicUnit=on
  Optimizer : Subsystem
  Product : Product
  Saturation : Saturate  UpperLimit=u_max_n6  LowerLimit=-u_max_n6
  Scope : Scope
  Sum : Sum  Inputs=-+|
  gain : Scope
  threshold : Constant  Value=th
  v : Scope
  y_an : Outport
  wires:
  threshold/1 -> MATLAB Function/2(th)
  Optimizer/1(v) -> Product/1, v/1
  u_sat/1 -> Optimizer/2(u_sat)
  MATLAB Function/1(G) -> gain/1, Product/2
  u/1 -> Optimizer/1(u)
  Annihilator/1(y_an) -> y_an/1
  Product/1 -> Annihilator/1(v)
  Saturation/1 -> Sum/1
  Sum/1 -> Scope/1, MATLAB Function/1(e)
  yc/1 -> Sum/2, Saturation/1

== system decentralized_trans/Sixth neighbour/Controller ==
  uc : Inport
  Clock1 : Clock
  Controller formation : Subsystem
  Controller line follow : Subsystem
  MATLAB Function : MATLAB Function  TreatAsAtomicUnit=on
  MATLAB Function1 : MATLAB Function  TreatAsAtomicUnit=on
  Scope : Scope
  t1 : Constant  Value=t1  VectorParams1D=off
  t2 : Constant  Value=t2  VectorParams1D=off
  t3 : Constant  Value=t3  VectorParams1D=off
  yc : Outport
  wires:
  uc/1 -> Controller formation/1(uc), Controller line follow/1(uc)
  Clock1/1 -> MATLAB Function1/1(t), MATLAB Function/2(t)
  Controller line follow/1(u) -> MATLAB Function/1(u_lf)
  Controller formation/1(u) -> MATLAB Function/3(u_f)
  t1/1 -> MATLAB Function1/2(t1), MATLAB Function/4(t1)
  t3/1 -> MATLAB Function1/4(t3), MATLAB Function/6(t3)
  MATLAB Function/1(yc) -> yc/1
  t2/1 -> MATLAB Function1/3(t2), MATLAB Function/5(t2)
  MATLAB Function1/1(y) -> Scope/1, Controller line follow/2(y), Controller formation/2(y)

== system decentralized_trans/Sixth neighbour/MRS ==
  u_MRS : Inport
  Constant : Constant  Value=b
  Integrator : Integrator  InitialCondition=p06
  Integrator1 : Integrator  InitialCondition=th02
  Integrator2 : Integrator  InitialCondition=phi02
  MATLAB Function : MATLAB Function  TreatAsAtomicUnit=on
  Scope : Scope
  Scope1 : Scope
  theta : ToWorkspace  VariableName=theta6  SampleTime=-1
  y : ToWorkspace  VariableName=y6  SampleTime=-1
  state : Outport
  wires:
  u_MRS/1 -> MATLAB Function/1(u)
  Constant/1 -> MATLAB Function/2(b)
  MATLAB Function/2(dth) -> Integrator1/1
  MATLAB Function/1(dp) -> Integrator/1
  Integrator1/1 -> MATLAB Function/3(th), Scope/1, theta/1
  MATLAB Function/3(dphi) -> Integrator2/1
  Integrator2/1 -> Scope1/1, MATLAB Function/4(phi)
  Integrator/1 -> y/1, state/1

== system decentralized_trans/Sixth neighbour/neighbour output ==
  p6 : Inport
  p5 : Inport  Port=2
  C : Gain  Gain=C2  Multiplication=Matrix(K*u) (u vector)
  C_id : Gain  Gain=C_id2  Multiplication=Matrix(K*u) (u vector)
  Clock : Clock
  MATLAB Function : MATLAB Function  TreatAsAtomicUnit=on
  MATLAB Function1 : MATLAB Function  TreatAsAtomicUnit=on
  t1 : Constant  Value=t1  VectorParams1D=off
  t2 : Constant  Value=t2  VectorParams1D=off
  t3 : Constant  Value=t3  VectorParams1D=off
  y_MRS : Outport
  state : Outport  Port=2
  wires:
  t2/1 -> MATLAB Function1/5(t2)
  C/1 -> MATLAB Function1/3(y_f)
  Clock/1 -> MATLAB Function1/2(t)
  t3/1 -> MATLAB Function1/6(t3)
  C_id/1 -> MATLAB Function1/1(y_lf)
  MATLAB Function1/1(y_MRS) -> y_MRS/1
  t1/1 -> MATLAB Function1/4(t1)
  MATLAB Function/1(yn) -> state/1, C/1, C_id/1
  p5/1 -> MATLAB Function/1(y1)
  p6/1 -> MATLAB Function/2(y2)

== system decentralized_trans/Sixth neighbour/ref generator ==
  t : Inport
  state : Inport  Port=2
  C1 : Gain  Gain=C2  Multiplication=Matrix(K*u) (u vector)
  C2 : Gain  Gain=C2  Multiplication=Matrix(K*u) (u vector)
  C_id : Gain  Gain=C_id2  Multiplication=Matrix(K*u) (u vector)
  Constant1 : Constant  Value=r_pd6  VectorParams1D=off
  Constant2 : Constant  Value=r_pd_sl6  VectorParams1D=off
  Constant3 : Constant  Value=dx2
  MATLAB Function : MATLAB Function  TreatAsAtomicUnit=on
  MATLAB Function1 : MATLAB Function  TreatAsAtomicUnit=on
  t1 : Constant  Value=t1  VectorParams1D=off
  t2 : Constant  Value=t2  VectorParams1D=off
  t3 : Constant  Value=t3  VectorParams1D=off
  r : Outport
  wires:
  t/1 -> MATLAB Function/1(t)
  t1/1 -> MATLAB Function/2(t1)
  t2/1 -> MATLAB Function/3(t2)
  t3/1 -> MATLAB Function/4(t3)
  Constant2/1 -> C2/1
  C2/1 -> MATLAB Function/6(r_pd2)
  Constant1/1 -> C1/1
  C1/1 -> MATLAB Function/5(r_pd)
  C_id/1 -> MATLAB Function/7(r_line)
  MATLAB Function/1(y) -> r/1
  Constant3/1 -> MATLAB Function1/1(dx)
  state/1 -> MATLAB Function1/2(state)
  MATLAB Function1/1(y) -> C_id/1

== system decentralized_trans/Third neighbour/Allocator ==
  u : Inport
  u_sat : Inport  Port=2
  yc : Inport  Port=3
  Annihilator : Subsystem
  MATLAB Function : MATLAB Function  TreatAsAtomicUnit=on
  Optimizer : Subsystem
  Product : Product
  Saturation : Saturate  UpperLimit=u_max_n3  LowerLimit=-u_max_n3
  Scope : Scope
  Sum : Sum  Inputs=-+|
  gain : Scope
  threshold : Constant  Value=th
  v : Scope
  y_an : Outport
  wires:
  threshold/1 -> MATLAB Function/2(th)
  Optimizer/1(v) -> Product/1, v/1
  u_sat/1 -> Optimizer/2(u_sat)
  MATLAB Function/1(G) -> gain/1, Product/2
  u/1 -> Optimizer/1(u)
  Annihilator/1(y_an) -> y_an/1
  Product/1 -> Annihilator/1(v)
  Saturation/1 -> Sum/1
  Sum/1 -> Scope/1, MATLAB Function/1(e)
  yc/1 -> Sum/2, Saturation/1

== system decentralized_trans/Third neighbour/Controller ==
  uc : Inport
  Clock1 : Clock
  Controller formation : Subsystem
  Controller line follow : Subsystem
  MATLAB Function : MATLAB Function  TreatAsAtomicUnit=on
  MATLAB Function1 : MATLAB Function  TreatAsAtomicUnit=on
  Scope : Scope
  t1 : Constant  Value=t1  VectorParams1D=off
  t2 : Constant  Value=t2  VectorParams1D=off
  t3 : Constant  Value=t3  VectorParams1D=off
  yc : Outport
  wires:
  uc/1 -> Controller formation/1(uc), Controller line follow/1(uc)
  Clock1/1 -> MATLAB Function1/1(t), MATLAB Function/2(t)
  Controller line follow/1(u) -> MATLAB Function/1(u_lf)
  Controller formation/1(u) -> MATLAB Function/3(u_f)
  t1/1 -> MATLAB Function1/2(t1), MATLAB Function/4(t1)
  t3/1 -> MATLAB Function1/4(t3), MATLAB Function/6(t3)
  MATLAB Function/1(yc) -> yc/1
  t2/1 -> MATLAB Function1/3(t2), MATLAB Function/5(t2)
  MATLAB Function1/1(y) -> Scope/1, Controller line follow/2(y), Controller formation/2(y)

== system decentralized_trans/Third neighbour/MRS ==
  u_MRS : Inport
  Constant : Constant  Value=b
  Integrator : Integrator  InitialCondition=p03
  Integrator1 : Integrator  InitialCondition=th02
  Integrator2 : Integrator  InitialCondition=phi02
  MATLAB Function : MATLAB Function  TreatAsAtomicUnit=on
  Scope : Scope
  Scope1 : Scope
  theta : ToWorkspace  VariableName=theta3  SampleTime=-1
  y : ToWorkspace  VariableName=y3  SampleTime=-1
  state : Outport
  wires:
  u_MRS/1 -> MATLAB Function/1(u)
  Constant/1 -> MATLAB Function/2(b)
  MATLAB Function/2(dth) -> Integrator1/1
  MATLAB Function/1(dp) -> Integrator/1
  Integrator1/1 -> MATLAB Function/3(th), Scope/1, theta/1
  MATLAB Function/3(dphi) -> Integrator2/1
  Integrator2/1 -> Scope1/1, MATLAB Function/4(phi)
  Integrator/1 -> y/1, state/1

== system decentralized_trans/Third neighbour/neighbour output ==
  p2 : Inport
  p3 : Inport  Port=2
  p4 : Inport  Port=3
  C : Gain  Gain=C3  Multiplication=Matrix(K*u) (u vector)
  C_id : Gain  Gain=C_id3  Multiplication=Matrix(K*u) (u vector)
  Clock : Clock
  MATLAB Function : MATLAB Function  TreatAsAtomicUnit=on
  MATLAB Function1 : MATLAB Function  TreatAsAtomicUnit=on
  t1 : Constant  Value=t1  VectorParams1D=off
  t2 : Constant  Value=t2  VectorParams1D=off
  t3 : Constant  Value=t3  VectorParams1D=off
  y_MRS : Outport
  state : Outport  Port=2
  wires:
  t2/1 -> MATLAB Function1/5(t2)
  C/1 -> MATLAB Function1/3(y_f)
  Clock/1 -> MATLAB Function1/2(t)
  t3/1 -> MATLAB Function1/6(t3)
  C_id/1 -> MATLAB Function1/1(y_lf)
  MATLAB Function1/1(y_MRS) -> y_MRS/1
  t1/1 -> MATLAB Function1/4(t1)
  MATLAB Function/1(yn) -> state/1, C/1, C_id/1
  p4/1 -> MATLAB Function/3(y3)
  p3/1 -> MATLAB Function/2(y2)
  p2/1 -> MATLAB Function/1(y1)

== system decentralized_trans/Third neighbour/ref generator ==
  t : Inport
  state : Inport  Port=2
  C1 : Gain  Gain=C3  Multiplication=Matrix(K*u) (u vector)
  C2 : Gain  Gain=C3  Multiplication=Matrix(K*u) (u vector)
  C_id : Gain  Gain=C_id3  Multiplication=Matrix(K*u) (u vector)
  Constant1 : Constant  Value=r_pd3  VectorParams1D=off
  Constant2 : Constant  Value=r_pd_sl3  VectorParams1D=off
  Constant3 : Constant  Value=dx3
  MATLAB Function : MATLAB Function  TreatAsAtomicUnit=on
  MATLAB Function1 : MATLAB Function  TreatAsAtomicUnit=on
  t1 : Constant  Value=t1  VectorParams1D=off
  t2 : Constant  Value=t2  VectorParams1D=off
  t3 : Constant  Value=t3  VectorParams1D=off
  r : Outport
  wires:
  t/1 -> MATLAB Function/1(t)
  t1/1 -> MATLAB Function/2(t1)
  t2/1 -> MATLAB Function/3(t2)
  t3/1 -> MATLAB Function/4(t3)
  Constant2/1 -> C2/1
  C2/1 -> MATLAB Function/6(r_pd2)
  Constant1/1 -> C1/1
  C1/1 -> MATLAB Function/5(r_pd)
  C_id/1 -> MATLAB Function/7(r_line)
  MATLAB Function/1(y) -> r/1
  Constant3/1 -> MATLAB Function1/1(dx)
  state/1 -> MATLAB Function1/2(state)
  MATLAB Function1/1(y) -> C_id/1

== system decentralized_trans/Fifth neighbour/Allocator/Annihilator ==
  v : Inport
  A_an : Gain  Gain=A_an3  Multiplication=Matrix(K*u) (u vector)
  B_an : Gain  Gain=B_an3  Multiplication=Matrix(K*u) (u vector)
  C_an : Gain  Gain=C_an3  Multiplication=Matrix(K*u) (u vector)
  D_an : Gain  Gain=D_an3  Multiplication=Matrix(K*u) (u vector)
  Integrator : Integrator  InitialCondition=xan03
  Sum : Sum  Inputs=|++
  Sum1 : Sum  Inputs=++|
  y_an1 : ToWorkspace  VariableName=yan5  SampleTime=-1
  y_an : Outport
  wires:
  Integrator/1 -> C_an/1, A_an/1
  B_an/1 -> Sum/2
  A_an/1 -> Sum/1
  v/1 -> D_an/1, B_an/1
  Sum/1 -> Integrator/1
  C_an/1 -> Sum1/2
  D_an/1 -> Sum1/1
  Sum1/1 -> y_an1/1, y_an/1

== system decentralized_trans/Fifth neighbour/Allocator/Optimizer ==
  u : Inport
  u_sat : Inport  Port=2
  C_opt : Gain  Gain=C_opt  Multiplication=Matrix(K*u) (u vector)
  Constant : Constant  Value=alpha
  Dan : Constant  Value=D_an3  VectorParams1D=off
  Integrator : Integrator  InitialCondition=xopt0
  Scope : Scope
  dx_opt : MATLAB Function  TreatAsAtomicUnit=on
  u_max : Constant  Value=u_max_n5
  v : Outport
  wires:
  dx_opt/1(dx_opt) -> Scope/1, Integrator/1
  C_opt/1 -> v/1
  Constant/1 -> dx_opt/1(alpha)
  Dan/1 -> dx_opt/2(D_an)
  u_max/1 -> dx_opt/3(u_max)
  u/1 -> dx_opt/4(u)
  u_sat/1 -> dx_opt/5(u_sat)
  Integrator/1 -> C_opt/1

== system decentralized_trans/Fifth neighbour/Controller/Controller formation ==
  uc : Inport
  y : Inport  Port=2
  Ac_mrs : Gain  Gain=Ac_mrs3  Multiplication=Matrix(K*u) (u vector)
  Bc_mrs : Gain  Gain=Bc_mrs3  Multiplication=Matrix(K*u) (u vector)
  Cc_mrs : Gain  Gain=Cc_mrs3  Multiplication=Matrix(K*u) (u vector)
  Dc_mrs : Gain  Gain=Dc_mrs3  Multiplication=Matrix(K*u) (u vector)
  Integrator : Integrator  ExternalReset=either  InitialCondition=xc03
  Sum : Sum  Inputs=|++
  Sum1 : Sum  Inputs=++|
  u : Outport
  wires:
  Bc_mrs/1 -> Sum1/1
  Cc_mrs/1 -> Sum/1
  uc/1 -> Bc_mrs/1, Dc_mrs/1
  Integrator/1 -> Ac_mrs/1, Cc_mrs/1
  Dc_mrs/1 -> Sum/2
  Sum/1 -> u/1
  Ac_mrs/1 -> Sum1/2
  Sum1/1 -> Integrator/1
  y/1 -> Integrator/2

== system decentralized_trans/Fifth neighbour/Controller/Controller line follow ==
  uc : Inport
  y : Inport  Port=2
  Ac_id : Gain  Gain=Ac_id3  Multiplication=Matrix(K*u) (u vector)
  Bc_id : Gain  Gain=Bc_id3  Multiplication=Matrix(K*u) (u vector)
  Cc_id : Gain  Gain=Cc_id3  Multiplication=Matrix(K*u) (u vector)
  Dc_id : Gain  Gain=Dc_id3  Multiplication=Matrix(K*u) (u vector)
  Integrator : Integrator  ExternalReset=either  InitialCondition=xc03
  Sum : Sum  Inputs=|++
  Sum1 : Sum  Inputs=++|
  u : Outport
  wires:
  Bc_id/1 -> Sum1/1
  Cc_id/1 -> Sum/1
  uc/1 -> Bc_id/1, Dc_id/1
  Integrator/1 -> Ac_id/1, Cc_id/1
  Dc_id/1 -> Sum/2
  Sum/1 -> u/1
  Ac_id/1 -> Sum1/2
  Sum1/1 -> Integrator/1
  y/1 -> Integrator/2

== system decentralized_trans/First neighbour/Allocator/Annihilator ==
  v : Inport
  A_an : Gain  Gain=A_an2  Multiplication=Matrix(K*u) (u vector)
  B_an : Gain  Gain=B_an2  Multiplication=Matrix(K*u) (u vector)
  C_an : Gain  Gain=C_an2  Multiplication=Matrix(K*u) (u vector)
  D_an : Gain  Gain=D_an2  Multiplication=Matrix(K*u) (u vector)
  Integrator : Integrator  InitialCondition=xan02
  Sum : Sum  Inputs=|++
  Sum1 : Sum  Inputs=++|
  y_an1 : ToWorkspace  VariableName=yan1  SampleTime=-1
  y_an : Outport
  wires:
  Integrator/1 -> C_an/1, A_an/1
  B_an/1 -> Sum/2
  A_an/1 -> Sum/1
  v/1 -> D_an/1, B_an/1
  Sum/1 -> Integrator/1
  C_an/1 -> Sum1/2
  D_an/1 -> Sum1/1
  Sum1/1 -> y_an1/1, y_an/1

== system decentralized_trans/First neighbour/Allocator/Optimizer ==
  u : Inport
  u_sat : Inport  Port=2
  C_opt : Gain  Gain=C_opt  Multiplication=Matrix(K*u) (u vector)
  Constant : Constant  Value=alpha
  Dan : Constant  Value=D_an2  VectorParams1D=off
  Integrator : Integrator  InitialCondition=xopt0
  Scope : Scope
  dx_opt : MATLAB Function  TreatAsAtomicUnit=on
  u_max : Constant  Value=u_max_n1
  v : Outport
  wires:
  dx_opt/1(dx_opt) -> Scope/1, Integrator/1
  C_opt/1 -> v/1
  Constant/1 -> dx_opt/1(alpha)
  Dan/1 -> dx_opt/2(D_an)
  u_max/1 -> dx_opt/3(u_max)
  u/1 -> dx_opt/4(u)
  u_sat/1 -> dx_opt/5(u_sat)
  Integrator/1 -> C_opt/1

== system decentralized_trans/First neighbour/Controller/Controller formation ==
  uc : Inport
  y : Inport  Port=2
  Ac_mrs : Gain  Gain=Ac_mrs2  Multiplication=Matrix(K*u) (u vector)
  Bc_mrs : Gain  Gain=Bc_mrs2  Multiplication=Matrix(K*u) (u vector)
  Cc_mrs : Gain  Gain=Cc_mrs2  Multiplication=Matrix(K*u) (u vector)
  Dc_mrs : Gain  Gain=Dc_mrs2  Multiplication=Matrix(K*u) (u vector)
  Integrator : Integrator  ExternalReset=either  InitialCondition=xc02
  Sum : Sum  Inputs=|++
  Sum1 : Sum  Inputs=++|
  u : Outport
  wires:
  Bc_mrs/1 -> Sum1/1
  Cc_mrs/1 -> Sum/1
  uc/1 -> Bc_mrs/1, Dc_mrs/1
  Integrator/1 -> Ac_mrs/1, Cc_mrs/1
  Dc_mrs/1 -> Sum/2
  Sum/1 -> u/1
  Ac_mrs/1 -> Sum1/2
  Sum1/1 -> Integrator/1
  y/1 -> Integrator/2

== system decentralized_trans/First neighbour/Controller/Controller line follow ==
  uc : Inport
  y : Inport  Port=2
  Ac_id : Gain  Gain=Ac_id2  Multiplication=Matrix(K*u) (u vector)
  Bc_id : Gain  Gain=Bc_id2  Multiplication=Matrix(K*u) (u vector)
  Cc_id : Gain  Gain=Cc_id2  Multiplication=Matrix(K*u) (u vector)
  Dc_id : Gain  Gain=Dc_id2  Multiplication=Matrix(K*u) (u vector)
  Integrator : Integrator  ExternalReset=either  InitialCondition=xc02
  Sum : Sum  Inputs=|++
  Sum1 : Sum  Inputs=++|
  u : Outport
  wires:
  Bc_id/1 -> Sum1/1
  Cc_id/1 -> Sum/1
  uc/1 -> Bc_id/1, Dc_id/1
  Integrator/1 -> Ac_id/1, Cc_id/1
  Dc_id/1 -> Sum/2
  Sum/1 -> u/1
  Ac_id/1 -> Sum1/2
  Sum1/1 -> Integrator/1
  y/1 -> Integrator/2

== system decentralized_trans/Fourth neighbour/Allocator/Annihilator ==
  v : Inport
  A_an : Gain  Gain=A_an3  Multiplication=Matrix(K*u) (u vector)
  B_an : Gain  Gain=B_an3  Multiplication=Matrix(K*u) (u vector)
  C_an : Gain  Gain=C_an3  Multiplication=Matrix(K*u) (u vector)
  D_an : Gain  Gain=D_an3  Multiplication=Matrix(K*u) (u vector)
  Integrator : Integrator  InitialCondition=xan03
  Sum : Sum  Inputs=|++
  Sum1 : Sum  Inputs=++|
  y_an1 : ToWorkspace  VariableName=yan4  SampleTime=-1
  y_an : Outport
  wires:
  Integrator/1 -> C_an/1, A_an/1
  B_an/1 -> Sum/2
  A_an/1 -> Sum/1
  v/1 -> D_an/1, B_an/1
  Sum/1 -> Integrator/1
  C_an/1 -> Sum1/2
  D_an/1 -> Sum1/1
  Sum1/1 -> y_an1/1, y_an/1

== system decentralized_trans/Fourth neighbour/Allocator/Optimizer ==
  u : Inport
  u_sat : Inport  Port=2
  C_opt : Gain  Gain=C_opt  Multiplication=Matrix(K*u) (u vector)
  Constant : Constant  Value=alpha
  Dan : Constant  Value=D_an3  VectorParams1D=off
  Integrator : Integrator  InitialCondition=xopt0
  Scope : Scope
  dx_opt : MATLAB Function  TreatAsAtomicUnit=on
  u_max : Constant  Value=u_max_n4
  v : Outport
  wires:
  dx_opt/1(dx_opt) -> Scope/1, Integrator/1
  C_opt/1 -> v/1
  Constant/1 -> dx_opt/1(alpha)
  Dan/1 -> dx_opt/2(D_an)
  u_max/1 -> dx_opt/3(u_max)
  u/1 -> dx_opt/4(u)
  u_sat/1 -> dx_opt/5(u_sat)
  Integrator/1 -> C_opt/1

== system decentralized_trans/Fourth neighbour/Controller/Controller formation ==
  uc : Inport
  y : Inport  Port=2
  Ac_mrs : Gain  Gain=Ac_mrs3  Multiplication=Matrix(K*u) (u vector)
  Bc_mrs : Gain  Gain=Bc_mrs3  Multiplication=Matrix(K*u) (u vector)
  Cc_mrs : Gain  Gain=Cc_mrs3  Multiplication=Matrix(K*u) (u vector)
  Dc_mrs : Gain  Gain=Dc_mrs3  Multiplication=Matrix(K*u) (u vector)
  Integrator : Integrator  ExternalReset=either  InitialCondition=xc03
  Sum : Sum  Inputs=|++
  Sum1 : Sum  Inputs=++|
  u : Outport
  wires:
  Bc_mrs/1 -> Sum1/1
  Cc_mrs/1 -> Sum/1
  uc/1 -> Bc_mrs/1, Dc_mrs/1
  Integrator/1 -> Ac_mrs/1, Cc_mrs/1
  Dc_mrs/1 -> Sum/2
  Sum/1 -> u/1
  Ac_mrs/1 -> Sum1/2
  Sum1/1 -> Integrator/1
  y/1 -> Integrator/2

== system decentralized_trans/Fourth neighbour/Controller/Controller line follow ==
  uc : Inport
  y : Inport  Port=2
  Ac_id : Gain  Gain=Ac_id3  Multiplication=Matrix(K*u) (u vector)
  Bc_id : Gain  Gain=Bc_id3  Multiplication=Matrix(K*u) (u vector)
  Cc_id : Gain  Gain=Cc_id3  Multiplication=Matrix(K*u) (u vector)
  Dc_id : Gain  Gain=Dc_id3  Multiplication=Matrix(K*u) (u vector)
  Integrator : Integrator  ExternalReset=either  InitialCondition=xc03
  Sum : Sum  Inputs=|++
  Sum1 : Sum  Inputs=++|
  u : Outport
  wires:
  Bc_id/1 -> Sum1/1
  Cc_id/1 -> Sum/1
  uc/1 -> Bc_id/1, Dc_id/1
  Integrator/1 -> Ac_id/1, Cc_id/1
  Dc_id/1 -> Sum/2
  Sum/1 -> u/1
  Ac_id/1 -> Sum1/2
  Sum1/1 -> Integrator/1
  y/1 -> Integrator/2

== system decentralized_trans/Second neighbour/Allocator/Annihilator ==
  v : Inport
  A_an : Gain  Gain=A_an3  Multiplication=Matrix(K*u) (u vector)
  B_an : Gain  Gain=B_an3  Multiplication=Matrix(K*u) (u vector)
  C_an : Gain  Gain=C_an3  Multiplication=Matrix(K*u) (u vector)
  D_an : Gain  Gain=D_an3  Multiplication=Matrix(K*u) (u vector)
  Integrator : Integrator  InitialCondition=xan03
  Sum : Sum  Inputs=|++
  Sum1 : Sum  Inputs=++|
  y_an1 : ToWorkspace  VariableName=yan2  SampleTime=-1
  y_an : Outport
  wires:
  Integrator/1 -> C_an/1, A_an/1
  B_an/1 -> Sum/2
  A_an/1 -> Sum/1
  v/1 -> D_an/1, B_an/1
  Sum/1 -> Integrator/1
  C_an/1 -> Sum1/2
  D_an/1 -> Sum1/1
  Sum1/1 -> y_an1/1, y_an/1

== system decentralized_trans/Second neighbour/Allocator/Optimizer ==
  u : Inport
  u_sat : Inport  Port=2
  C_opt : Gain  Gain=C_opt  Multiplication=Matrix(K*u) (u vector)
  Constant : Constant  Value=alpha
  Dan : Constant  Value=D_an3  VectorParams1D=off
  Integrator : Integrator  InitialCondition=xopt0
  Scope : Scope
  dx_opt : MATLAB Function  TreatAsAtomicUnit=on
  u_max : Constant  Value=u_max_n2
  v : Outport
  wires:
  dx_opt/1(dx_opt) -> Scope/1, Integrator/1
  C_opt/1 -> v/1
  Constant/1 -> dx_opt/1(alpha)
  Dan/1 -> dx_opt/2(D_an)
  u_max/1 -> dx_opt/3(u_max)
  u/1 -> dx_opt/4(u)
  u_sat/1 -> dx_opt/5(u_sat)
  Integrator/1 -> C_opt/1

== system decentralized_trans/Second neighbour/Controller/Controller formation ==
  uc : Inport
  y : Inport  Port=2
  Ac_mrs : Gain  Gain=Ac_mrs3  Multiplication=Matrix(K*u) (u vector)
  Bc_mrs : Gain  Gain=Bc_mrs3  Multiplication=Matrix(K*u) (u vector)
  Cc_mrs : Gain  Gain=Cc_mrs3  Multiplication=Matrix(K*u) (u vector)
  Dc_mrs : Gain  Gain=Dc_mrs3  Multiplication=Matrix(K*u) (u vector)
  Integrator : Integrator  ExternalReset=either  InitialCondition=xc03
  Sum : Sum  Inputs=|++
  Sum1 : Sum  Inputs=++|
  u : Outport
  wires:
  Bc_mrs/1 -> Sum1/1
  Cc_mrs/1 -> Sum/1
  uc/1 -> Bc_mrs/1, Dc_mrs/1
  Integrator/1 -> Ac_mrs/1, Cc_mrs/1
  Dc_mrs/1 -> Sum/2
  Sum/1 -> u/1
  Ac_mrs/1 -> Sum1/2
  Sum1/1 -> Integrator/1
  y/1 -> Integrator/2

== system decentralized_trans/Second neighbour/Controller/Controller line follow ==
  uc : Inport
  y : Inport  Port=2
  Ac_id : Gain  Gain=Ac_id3  Multiplication=Matrix(K*u) (u vector)
  Bc_id : Gain  Gain=Bc_id3  Multiplication=Matrix(K*u) (u vector)
  Cc_id : Gain  Gain=Cc_id3  Multiplication=Matrix(K*u) (u vector)
  Dc_id : Gain  Gain=Dc_id3  Multiplication=Matrix(K*u) (u vector)
  Integrator : Integrator  ExternalReset=either  InitialCondition=xc03
  Sum : Sum  Inputs=|++
  Sum1 : Sum  Inputs=++|
  u : Outport
  wires:
  Bc_id/1 -> Sum1/1
  Cc_id/1 -> Sum/1
  uc/1 -> Bc_id/1, Dc_id/1
  Integrator/1 -> Ac_id/1, Cc_id/1
  Dc_id/1 -> Sum/2
  Sum/1 -> u/1
  Ac_id/1 -> Sum1/2
  Sum1/1 -> Integrator/1
  y/1 -> Integrator/2

== system decentralized_trans/Sixth neighbour/Allocator/Annihilator ==
  v : Inport
  A_an : Gain  Gain=A_an2  Multiplication=Matrix(K*u) (u vector)
  B_an : Gain  Gain=B_an2  Multiplication=Matrix(K*u) (u vector)
  C_an : Gain  Gain=C_an2  Multiplication=Matrix(K*u) (u vector)
  D_an : Gain  Gain=D_an2  Multiplication=Matrix(K*u) (u vector)
  Integrator : Integrator  InitialCondition=xan02
  Sum : Sum  Inputs=|++
  Sum1 : Sum  Inputs=++|
  y_an1 : ToWorkspace  VariableName=yan6  SampleTime=-1
  y_an : Outport
  wires:
  Integrator/1 -> C_an/1, A_an/1
  B_an/1 -> Sum/2
  A_an/1 -> Sum/1
  v/1 -> D_an/1, B_an/1
  Sum/1 -> Integrator/1
  C_an/1 -> Sum1/2
  D_an/1 -> Sum1/1
  Sum1/1 -> y_an1/1, y_an/1

== system decentralized_trans/Sixth neighbour/Allocator/Optimizer ==
  u : Inport
  u_sat : Inport  Port=2
  C_opt : Gain  Gain=C_opt  Multiplication=Matrix(K*u) (u vector)
  Constant : Constant  Value=alpha
  Dan : Constant  Value=D_an2  VectorParams1D=off
  Integrator : Integrator  InitialCondition=xopt0
  Scope : Scope
  dx_opt : MATLAB Function  TreatAsAtomicUnit=on
  u_max : Constant  Value=u_max_n6
  v : Outport
  wires:
  dx_opt/1(dx_opt) -> Scope/1, Integrator/1
  C_opt/1 -> v/1
  Constant/1 -> dx_opt/1(alpha)
  Dan/1 -> dx_opt/2(D_an)
  u_max/1 -> dx_opt/3(u_max)
  u/1 -> dx_opt/4(u)
  u_sat/1 -> dx_opt/5(u_sat)
  Integrator/1 -> C_opt/1

== system decentralized_trans/Sixth neighbour/Controller/Controller formation ==
  uc : Inport
  y : Inport  Port=2
  Ac_mrs : Gain  Gain=Ac_mrs2  Multiplication=Matrix(K*u) (u vector)
  Bc_mrs : Gain  Gain=Bc_mrs2  Multiplication=Matrix(K*u) (u vector)
  Cc_mrs : Gain  Gain=Cc_mrs2  Multiplication=Matrix(K*u) (u vector)
  Dc_mrs : Gain  Gain=Dc_mrs2  Multiplication=Matrix(K*u) (u vector)
  Integrator : Integrator  ExternalReset=either  InitialCondition=xc02
  Sum : Sum  Inputs=|++
  Sum1 : Sum  Inputs=++|
  u : Outport
  wires:
  Bc_mrs/1 -> Sum1/1
  Cc_mrs/1 -> Sum/1
  uc/1 -> Bc_mrs/1, Dc_mrs/1
  Integrator/1 -> Ac_mrs/1, Cc_mrs/1
  Dc_mrs/1 -> Sum/2
  Sum/1 -> u/1
  Ac_mrs/1 -> Sum1/2
  Sum1/1 -> Integrator/1
  y/1 -> Integrator/2
